simulink model "acquisition"  (Simulink 5.0)
settings: Solver=ode45  StartTime=0.0  StopTime=inf  RelTol=1e-3
libraries: dspwin32 x2, dspsnks4 x1
settings Model: LastModifiedBy=Miky

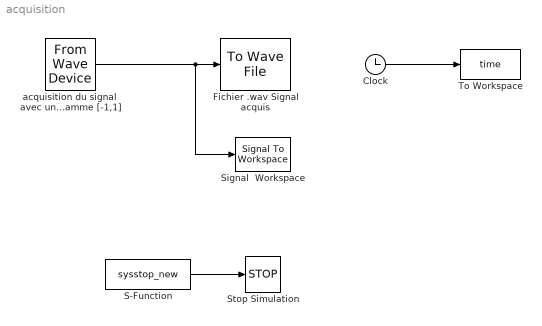
== system acquisition ==
  Clock : Clock
      settings: Decimation=10
  Fichier .wav Signal acquis : dspwin32/To Wave File  filename=voix.wav  sampleWidth=32  MinNumSamples=256
  S-Function : S-Function  FunctionName=sysstop_new
  Signal  Workspace : dspsnks4/Signal To Workspace  VariableName=voix  FrameMode=Concatenate frames (2-D array)
  Stop Simulation : Stop
  To Workspace : ToWorkspace  VariableName=time  SampleTime=-1  SaveFormat=StructureWithTime
      settings: MaxDataPoints=1
  acquisition du signal  avec un microphone Gamme [-1,1] : dspwin32/From Wave Device  SampleRate=8000  UserRate=16000  SampleWidth=8  Stereo=off  SamplesPerFrame=80  QueueDuration=1  useDefaultDevice=on  userDeviceID=Realtek AC97 Audio  dType=Double
  wires:
  acquisition du signal  avec un microphone Gamme [-1,1]/1 -> Fichier .wav Signal acquis/1, Signal  Workspace/1
  S-Function/1 -> Stop Simulation/1
  Clock/1 -> To Workspace/1
